simulink model "Simulink_DC_MG_4DGs_4Lines"  (R2024a)
settings: Solver=VariableStepAuto  StartTime=0.0  StopTime=10  RelTol=1e-3
values from neighbouring files (symbols this model uses):
  Is = Is_new    [implementLemma4_iterative.m]    (also in implementTheorem1.m = value(Is))
  numOfDGs = size(B_il,1)    [centralizedLocalControlDesign.m]    (also in globalControlDesign.m; verifyControlConditions.m)
undefined symbols (not defined in the file or in its folder): CCL_Coefficient, CPL_activation, DC_Activation, DG, K, LC_Activation, Line, PlugIn, PlugOut, SS_Activation, V_nom, V_ref
libraries: spsSeriesRLCBranchLib x28, spsCurrentMeasurementLib x12, spsControlledCurrentSourceLib x8, spsVoltageMeasurementLib x8, simulink x4, spsIdealSwitchLib x4, spsStairGeneratorLib x4, spsDCVoltageSourceLib x4, spsDiodeLib x4, spsIGBTLib x4, spspowerguiLib x1
(part 2 of 2)

== system Simulink_DC_MG_4DGs_4Lines/Local and Global Controller /Subsystem3/Steady State Control Activation ==
  Clock : Clock
  Constant1 : Constant  Value=SS_Activation
  Relational Operator : RelationalOperator  OutDataTypeStr=boolean  RndMeth=Simplest  InputSameDT=off
  Out1 : Outport  VectorParamsAs1DForOutWhenUnconnected=off
  wires:
  Clock/1 -> Relational Operator/1
  Relational Operator/1 -> Out1/1
  Constant1/1 -> Relational Operator/2

== system Simulink_DC_MG_4DGs_4Lines/Local and Global Controller /Subsystem3/Subsystem2 ==
  u : Inport
  0.05 : Gain
  Relational Operator : RelationalOperator  OutDataTypeStr=boolean  InputSameDT=off
  Scope : Scope  NumInputPorts=2
  Scope2 : Scope
  Triangle1 : simulink/Sources/Repeating Sequence  rep_seq_t=[0 40e-5 80e-5]  rep_seq_y=[0 1 0]
  PWM : Outport
  wires:
  0.05/1 -> Relational Operator/1, Scope/1
  Triangle1/1 -> Relational Operator/2, Scope/2
  u/1 -> 0.05/1
  Relational Operator/1 -> PWM/1, Scope2/1
